simulink model "ECM"  (R2025b)
settings: Solver=VariableStepAuto  StartTime=0.0  StopTime=60000  MaxStep=1  RelTol=1e-3
values from neighbouring files (symbols this model uses):
  AH = 2.5    [DataECM.sldd]
  C1_table = 14.038662996835537 14.038662996835537 14.038662996835537 14.038662996835537 14.038662996835537 14.038662996835537 14.038662996835537 14.038662996835537 14.038662996835537 13.716152424824331 13.70780042 13.70767275 15.4876125 15.52608855 15.37737691983936 15.37737691983936 15.37737691983936 15.37737691983936 15.37737691983936 15.37737691983936 15.37737691983936 14.359723373671073 14.359723373671073    [DataECM.sldd]
  C2_table = 1352.6468827825752 1352.6468827825752 1352.6468827825752 1352.6468827825752 1352.6468827825752 1352.6468827825752 1352.6468827825752 1352.6468827825752 1352.6468827825752 1358.3962866279012 1361.204699 1361.204668 1489.818558 1489.818563 1453.2108509645884 1453.2108509645884 1453.2108509645884 1453.2108509645884 1453.2108509645884 1453.2108509645884 1453.2108509645884 1344.0891535651501 1344.08915    [DataECM.sldd]
  Crate_bp = 0.25 0.5 1.0 2.0 5.0 8.0 10.0 15.0    [DataECM.sldd]
  OCV = 3.077 3.1749 3.1967 3.2132 3.2338 3.2636 3.2838 3.286 3.2892 3.3039 3.3274 3.3292 3.3316 3.4469    [DataECM.sldd]
  R0_table = 0.0013697001953677269 0.0013697001953677269 0.0013697001953677269 0.0013697001953677269 0.0013697001953677269 0.0013697001953677269 0.0013697001953677269 0.0013697001953677269 0.0013697001953677269 0.00047575923642928091 0.0003277717761 0.0003277717761 0.0003841075501 0.0003841075501 0.00047396535261650448 0.00047396535261650448 0.00047396535261650448 0.00047396535261650448 0.00047396535261650448    [DataECM.sldd]
  R1_table = 0.0084007312474261228 0.0084007312474261228 0.0084007312474261228 0.0084007312474261228 0.0084007312474261228 0.0084007312474261228 0.0084007312474261228 0.0084007312474261228 0.0084007312474261228 0.0084955040256046478 0.008506708375 0.008525806321 0.009190588347 0.009184896157 0.009050179402327798 0.009050179402327798 0.009050179402327798 0.009050179402327798 0.009050179402327798 0.0090501794023    [DataECM.sldd]
  R2_table = 0.015106319088391846 0.015106319088391846 0.015106319088391846 0.015106319088391846 0.015106319088391846 0.015106319088391846 0.015106319088391846 0.015106319088391846 0.015106319088391846 0.014877593755183665 0.01478557796 0.01478557796 0.01454122871 0.01454122871 0.014670782061069287 0.014670782061069287 0.014670782061069287 0.014670782061069287 0.014670782061069287 0.014670782061069287 0.014670    [DataECM.sldd]
  SOC0 = 0.5    [DataECM.sldd]
  SOC_bp = 0.0 5.0 10.0 15.0 20.0 25.0 30.0 35.0 40.0 45.0 50.0 55.0 60.0 65.0 70.0 75.0 80.0 85.0 90.0 95.0 100.0    [DataECM.sldd]
  SOCT = 2.5 5.0 10.0 15.0 20.0 30.0 40.0 50.0 60.0 70.0 80.0 90.0 95.0 100.0    [DataECM.sldd]
  Ts = 1.0    [DataECM.sldd]
settings Model: DataDictionary=DataECM.sldd  LastModifiedBy=yashn

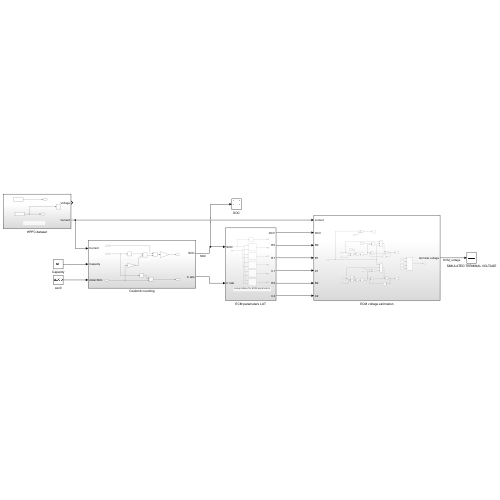
[thumbnail: Simulink's stored preview of the top-level diagram]
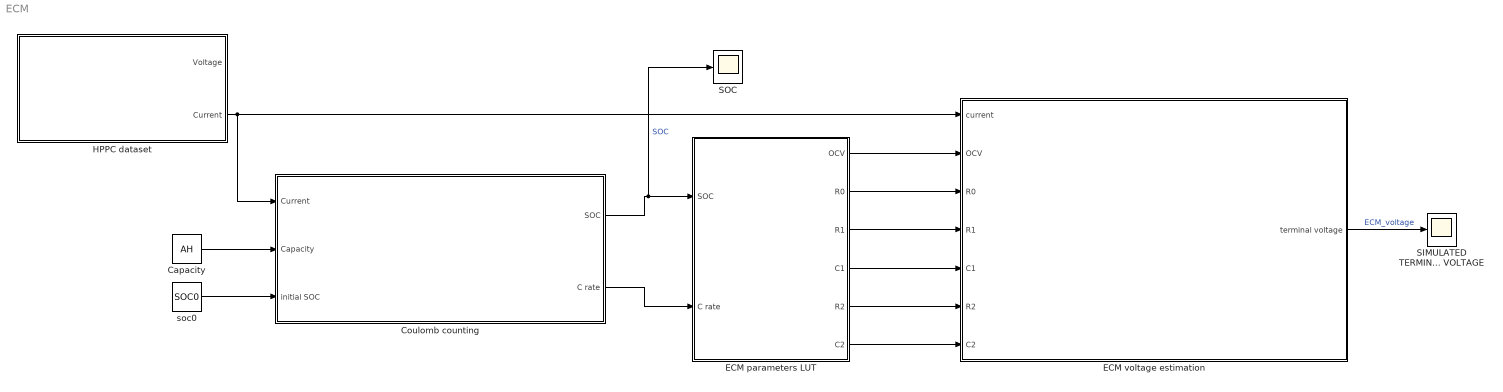
== system ECM ==
  Capacity : Constant  Value=AH
  Coulomb counting : Subsystem
  ECM parameters LUT : Subsystem
  ECM voltage estimation : Subsystem
  HPPC dataset : Subsystem
  SIMULATED TERMINAL VOLTAGE : Scope
      settings: ActiveDisplayYMinimum=2.8354164118859808  ActiveDisplayYMaximum=3.5707107115227941  YLabel=Voltage(v)
  SOC : Scope
      settings: ActiveDisplayYMinimum=43.511973394337872  ActiveDisplayYMaximum=67.653885031469827  YLabel=SOC(%)
  soc0 : Constant  Value=SOC0
  wires:
  ECM parameters LUT/4(C1) -> ECM voltage estimation/5(C1)
  Capacity/1 -> Coulomb counting/2(Capacity)
  ECM parameters LUT/5(R2) -> ECM voltage estimation/6(R2)
  ECM parameters LUT/6(C2) -> ECM voltage estimation/7(C2)
  ECM parameters LUT/3(R1) -> ECM voltage estimation/4(R1)
  Coulomb counting/2(C rate) -> ECM parameters LUT/2(C rate)
  Coulomb counting/1(SOC) -> SOC/1, ECM parameters LUT/1(SOC)  "SOC"
  ECM parameters LUT/2(R0) -> ECM voltage estimation/3(R0)
  soc0/1 -> Coulomb counting/3(initial SOC)
  HPPC dataset/2(Current) -> Coulomb counting/1(Current), ECM voltage estimation/1(current)
  ECM parameters LUT/1(OCV) -> ECM voltage estimation/2(OCV)
  ECM voltage estimation/1(terminal voltage) -> SIMULATED TERMINAL VOLTAGE/1  "ECM_voltage"

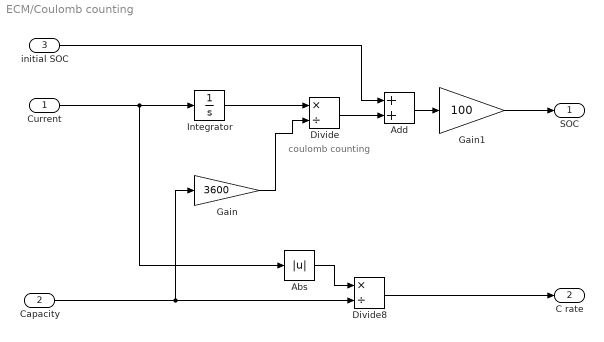
== system ECM/Coulomb counting ==
  note: coulomb counting
  Current : Inport
  Capacity : Inport  Port=2
  initial SOC : Inport  Port=3
  Abs : Abs  SaturateOnIntegerOverflow=off
  Add : Sum
  Divide : Product  Inputs=*/
  Divide8 : Product  Inputs=*/
  Gain : Gain  Gain=3600
  Gain1 : Gain  Gain=100
  Integrator : Integrator
  SOC : Outport
  C rate : Outport  Port=2
  wires:
  Gain1/1 -> SOC/1
  initial SOC/1 -> Add/1
  Add/1 -> Gain1/1
  Divide/1 -> Add/2
  Divide8/1 -> C rate/1
  Capacity/1 -> Gain/1, Divide8/2
  Current/1 -> Abs/1, Integrator/1
  Abs/1 -> Divide8/1
  Gain/1 -> Divide/2
  Integrator/1 -> Divide/1

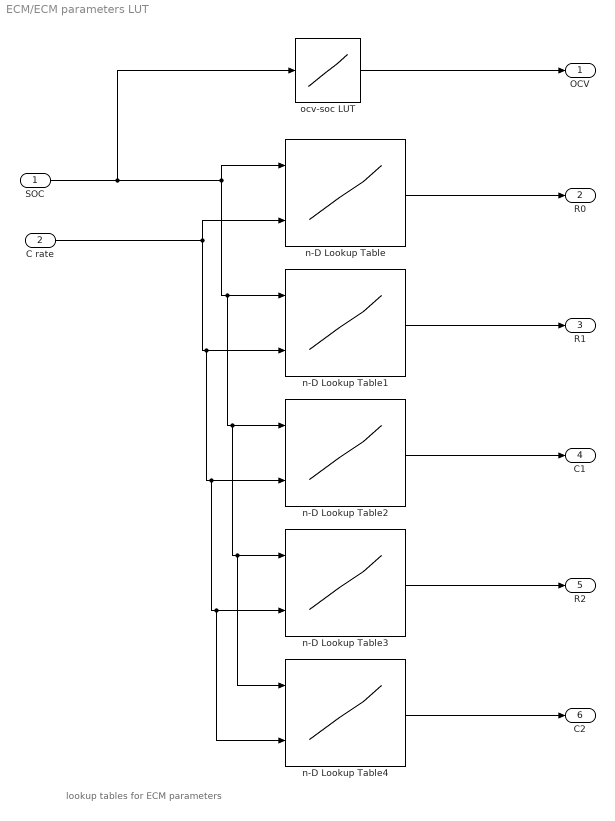
== system ECM/ECM parameters LUT ==
  note: lookup tables for ECM parameters
  SOC : Inport
  C rate : Inport  Port=2
  n-D Lookup Table : Lookup_n-D  BreakpointsForDimension1=SOC_bp  BreakpointsForDimension2=Crate_bp  BreakpointsForDimension3=[5, 7]  Table=R0_table  InterpMethod=Linear Lagrange  InternalRulePriority=Speed  RndMeth=Simplest
      settings: InputPortMap=u0,u1
  n-D Lookup Table1 : Lookup_n-D  BreakpointsForDimension1=SOC_bp  BreakpointsForDimension2=Crate_bp  BreakpointsForDimension3=[5, 7]  Table=R1_table  InterpMethod=Linear Lagrange  InternalRulePriority=Speed  RndMeth=Simplest
      settings: InputPortMap=u0,u1
  n-D Lookup Table2 : Lookup_n-D  BreakpointsForDimension1=SOC_bp  BreakpointsForDimension2=Crate_bp  BreakpointsForDimension3=[5, 7]  Table=C1_table  InterpMethod=Linear Lagrange  InternalRulePriority=Speed  RndMeth=Simplest
      settings: InputPortMap=u0,u1
  n-D Lookup Table3 : Lookup_n-D  BreakpointsForDimension1=SOC_bp  BreakpointsForDimension2=Crate_bp  BreakpointsForDimension3=[5, 7]  Table=R2_table  InterpMethod=Linear Lagrange  InternalRulePriority=Speed  RndMeth=Simplest
      settings: InputPortMap=u0,u1
  n-D Lookup Table4 : Lookup_n-D  BreakpointsForDimension1=SOC_bp  BreakpointsForDimension2=Crate_bp  BreakpointsForDimension3=[5, 7]  Table=C2_table  InterpMethod=Linear Lagrange  InternalRulePriority=Speed  RndMeth=Simplest
      settings: InputPortMap=u0,u1
  ocv-soc LUT : Lookup_n-D  NumberOfTableDimensions=1  BreakpointsForDimension1=SOCT  Table=OCV  InternalRulePriority=Speed  RndMeth=Simplest
  OCV : Outport
  R0 : Outport  Port=2
  R1 : Outport  Port=3
  C1 : Outport  Port=4
  R2 : Outport  Port=5
  C2 : Outport  Port=6
  wires:
  ocv-soc LUT/1 -> OCV/1
  C rate/1 -> n-D Lookup Table4/2, n-D Lookup Table3/2, n-D Lookup Table2/2, n-D Lookup Table1/2, n-D Lookup Table/2
  SOC/1 -> ocv-soc LUT/1, n-D Lookup Table/1, n-D Lookup Table4/1, n-D Lookup Table3/1, n-D Lookup Table2/1, n-D Lookup Table1/1
  n-D Lookup Table1/1 -> R1/1
  n-D Lookup Table/1 -> R0/1
  n-D Lookup Table2/1 -> C1/1
  n-D Lookup Table3/1 -> R2/1
  n-D Lookup Table4/1 -> C2/1

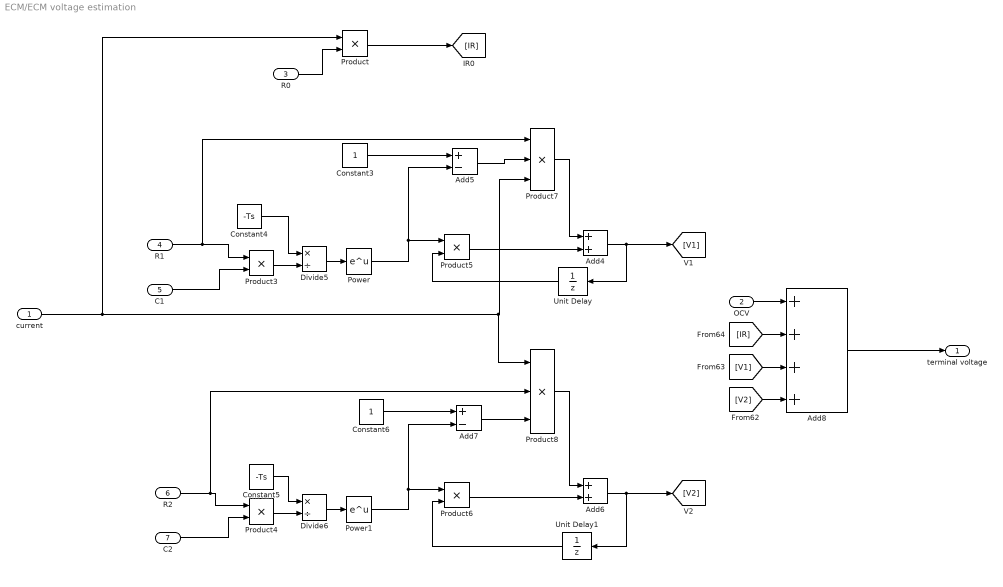
== system ECM/ECM voltage estimation ==
  current : Inport
  OCV : Inport  Port=2
  R0 : Inport  Port=3
  R1 : Inport  Port=4
  C1 : Inport  Port=5
  R2 : Inport  Port=6
  C2 : Inport  Port=7
  Add4 : Sum
  Add5 : Sum  Inputs=+-
  Add6 : Sum
  Add7 : Sum  Inputs=+-
  Add8 : Sum  Inputs=++++
  Constant3 : Constant
  Constant4 : Constant  Value=-Ts
  Constant5 : Constant  Value=-Ts
  Constant6 : Constant
  Divide5 : Product  Inputs=*/
  Divide6 : Product  Inputs=*/
  Power : Math
  Power1 : Math
  Product{,3..6} (5 alike) : Product
  Product7 : Product  Inputs=3
  Product8 : Product  Inputs=3
  Unit Delay : UnitDelay  SampleTime=-1  HasFrameUpgradeWarning=on
  Unit Delay1 : UnitDelay  SampleTime=-1  HasFrameUpgradeWarning=on
  terminal voltage : Outport
  wires:
  Divide6/1 -> Power1/1
  C1/1 -> Product3/2
  Add4/1 -> [V1], Unit Delay/1
  Product5/1 -> Add4/2
  Product7/1 -> Add4/1
  Product/1 -> [IR]
  Product4/1 -> Divide6/2
  Constant6/1 -> Add7/1
  Divide5/1 -> Power/1
  Power1/1 -> Product6/1, Add7/2
  Product3/1 -> Divide5/2
  Constant5/1 -> Divide6/1
  R1/1 -> Product7/1, Product3/1
  [V1] -> Add8/3
  [V2] -> Add8/4
  Unit Delay1/1 -> Product6/2
  OCV/1 -> Add8/1
  Add6/1 -> [V2], Unit Delay1/1
  [IR] -> Add8/2
  R0/1 -> Product/2
  current/1 -> Product/1, Product8/1, Product7/3
  Constant3/1 -> Add5/1
  R2/1 -> Product8/2, Product4/1
  Product8/1 -> Add6/1
  Product6/1 -> Add6/2
  Constant4/1 -> Divide5/1
  Add5/1 -> Product7/2
  Power/1 -> Product5/1, Add5/2
  C2/1 -> Product4/2
  Unit Delay/1 -> Product5/2
  Add8/1 -> terminal voltage/1
  Add7/1 -> Product8/3

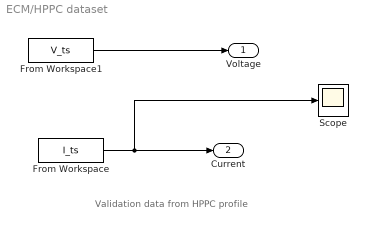
== system ECM/HPPC dataset ==
  note: Validation data from HPPC profile
  From Workspace : FromWorkspace  VariableName=I_ts  OutDataTypeStr=double  SampleTime=-1
  From Workspace1 : FromWorkspace  VariableName=V_ts  OutDataTypeStr=double  SampleTime=-1
  Scope : Scope
      settings: ActiveDisplayYMinimum=-46.256130152343744  ActiveDisplayYMaximum=29.210126097656257  DataLoggingVariableName=ScopeData2
  Voltage : Outport
  Current : Outport  Port=2
  wires:
  From Workspace1/1 -> Voltage/1
  From Workspace/1 -> Current/1, Scope/1
